simulink model "BLDC_speed_control"  (Simulink 8.1)
settings: Solver=ode45  StartTime=0.0  StopTime=1  RelTol=1e-3
InitFcn:
  | clc;
StopFcn:
  | clc;
undefined symbols (not defined in the file): emfg, Ts
libraries: simulink x6, powerlib x6, powerlib_extras x1
Description:
  | This simulink model simulates the speed control of permanent magnet
  | brush less DC motor. Complete dynamic model of brush-less DC motor
  | was developed and simulated. Conventional PI controller was employed
  | for speed loop.
  | 
  | Syed Abdul Rahman Kashif
  | EED, UET, Lahore
settings Model: Creator=AbdulRahman  LastModifiedBy=Sony
settings DataIOCC: SignalLoggingSaveFormat=Dataset
settings DebuggingCC: FcnCallInpInsideContextMsg=EnableAllAsError
settings GRTTargetCC: CombineOutputUpdateFcns=on  GRTInterface=off

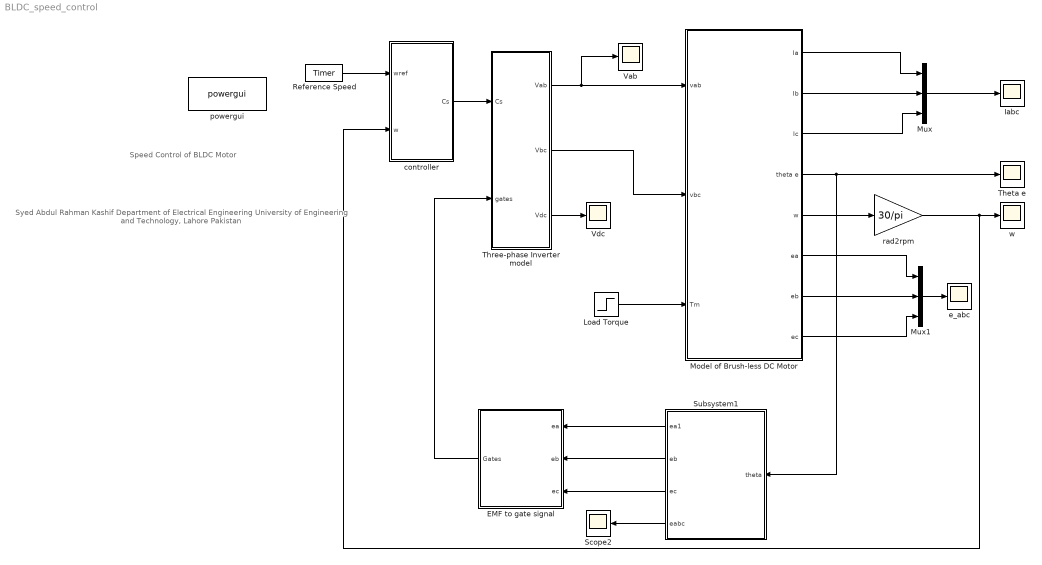
== system BLDC_speed_control ==
  note: Syed Abdul Rahman Kashif
      | Department of Electrical Engineering
      | University of Engineering and Technology, Lahore
      | Pakistan
  note: Speed Control of BLDC Motor
  EMF to gate signal : Subsystem
  Iabc : Scope
      settings: YMin=-0.3  YMax=0.3  SaveName=ScopeData4
  Load Torque : Step  Time=0.2  After=2  SampleTime=0
  Model of Brush-less DC Motor : Subsystem
  Mux : Mux  Inputs=3
  Mux1 : Mux  Inputs=3
  Reference Speed : powerlib_extras/Control  Blocks/Timer  t=[0 0.5]  e=[2000 1000]
  Scope2 : Scope
      settings: TimeRange=0.2  YMin=-2  YMax=2  SaveName=ScopeData2
  Subsystem1 : Subsystem
  Theta e : Scope
      settings: YMin=1.00059  YMax=1.00067
  Three-phase Inverter model : Subsystem
  Vab : Scope
      settings: TimeRange=0.2  YMin=-10000  YMax=10000  SaveName=ScopeData3
  Vdc : Scope
      settings: SaveName=ScopeData5
  controller : Subsystem
  e_abc : Scope
      settings: TimeRange=0.0001172995862488424  YMin=-150  YMax=150  SaveName=ScopeData6
  powergui : powerlib/powergui  Priority=2  SimulationMode=Continuous  SolverType=Tustin  SampleTime=Ts  frequency=60  SPID=off  DisableSnubberDevices=off  DisableRonSwitches=off  DisableVfSwitches=off  SwTol=0  Interpol=off  DisplayEquations=off  frequencyindice=0  Pbase=100e6  ErrMax=1e-4  Iterations=50  UnitsV=kV  UnitsW=MW  FunctionMessages=off  echomessages=off  HookPort=off  EnableUseOfTLC=off  x0status=blocks  RestoreLinks=warning  ResistiveCurrentMeasurement=off  Frange=[0:2:500]  Ylog=off  Xlog=on  ShowGrid=off  save=off  variable=ZData  ZoomFFT=on  StartTime=0.0  cycles=1  DisplayStyle=1  fundamental=60  FreqAxis=off  MaxFrequency=1000  frequencyindicesteady=1  RmsSteady=1  display=off  Ts=0  methode=off
  rad2rpm : Gain  Gain=30/pi
  w : Scope
      settings: TimeRange=0.4  YMin=0  YMax=2500
  wires:
  controller/1(Cs) -> Three-phase Inverter model/1(Cs)
  Three-phase Inverter model/2(Vbc) -> Model of Brush-less DC Motor/2(vbc)
  Three-phase Inverter model/3(Vdc) -> Vdc/1
  EMF to gate signal/1(Gates) -> Three-phase Inverter model/2(gates)
  Subsystem1/1(ea1) -> EMF to gate signal/1(ea)
  Subsystem1/2(eb) -> EMF to gate signal/2(eb)
  Subsystem1/3(ec) -> EMF to gate signal/3(ec)
  Model of Brush-less DC Motor/4(theta e) -> Theta e/1, Subsystem1/1(theta)
  Load Torque/1 -> Model of Brush-less DC Motor/3(Tm)
  Model of Brush-less DC Motor/2(Ib) -> Mux/2
  Model of Brush-less DC Motor/3(Ic) -> Mux/3
  Model of Brush-less DC Motor/6(ea) -> Mux1/1
  Model of Brush-less DC Motor/7(eb) -> Mux1/2
  Model of Brush-less DC Motor/8(ec) -> Mux1/3
  Mux1/1 -> e_abc/1
  Subsystem1/4(eabc) -> Scope2/1
  Model of Brush-less DC Motor/5(w) -> rad2rpm/1
  rad2rpm/1 -> controller/2(w), w/1
  Model of Brush-less DC Motor/1(Ia) -> Mux/1
  Mux/1 -> Iabc/1
  Reference Speed/1 -> controller/1(wref)
  Three-phase Inverter model/1(Vab) -> Model of Brush-less DC Motor/1(vab), Vab/1

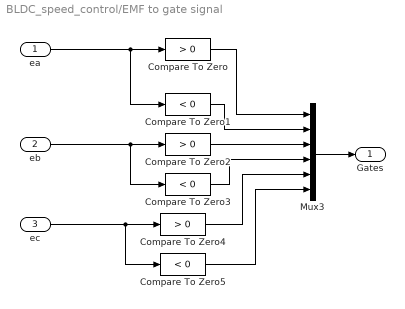
== system BLDC_speed_control/EMF to gate signal ==
  ea : Inport
  eb : Inport  Port=2
  ec : Inport  Port=3
  Compare To Zero : simulink/Logic and Bit Operations/Compare To Zero  relop=>  OutDataTypeStr=boolean  ZeroCross=off
  Compare To Zero1 : simulink/Logic and Bit Operations/Compare To Zero  relop=<  OutDataTypeStr=boolean  ZeroCross=off
  Compare To Zero2 : simulink/Logic and Bit Operations/Compare To Zero  relop=>  OutDataTypeStr=boolean  ZeroCross=off
  Compare To Zero3 : simulink/Logic and Bit Operations/Compare To Zero  relop=<  OutDataTypeStr=boolean  ZeroCross=off
  Compare To Zero4 : simulink/Logic and Bit Operations/Compare To Zero  relop=>  OutDataTypeStr=boolean  ZeroCross=off
  Compare To Zero5 : simulink/Logic and Bit Operations/Compare To Zero  relop=<  OutDataTypeStr=boolean  ZeroCross=off
  Mux3 : Mux  Inputs=6
  Gates : Outport
  wires:
  Mux3/1 -> Gates/1
  ea/1 -> Compare To Zero/1, Compare To Zero1/1
  eb/1 -> Compare To Zero2/1, Compare To Zero3/1
  ec/1 -> Compare To Zero4/1, Compare To Zero5/1
  Compare To Zero/1 -> Mux3/1
  Compare To Zero1/1 -> Mux3/2
  Compare To Zero2/1 -> Mux3/3
  Compare To Zero3/1 -> Mux3/4
  Compare To Zero4/1 -> Mux3/5
  Compare To Zero5/1 -> Mux3/6

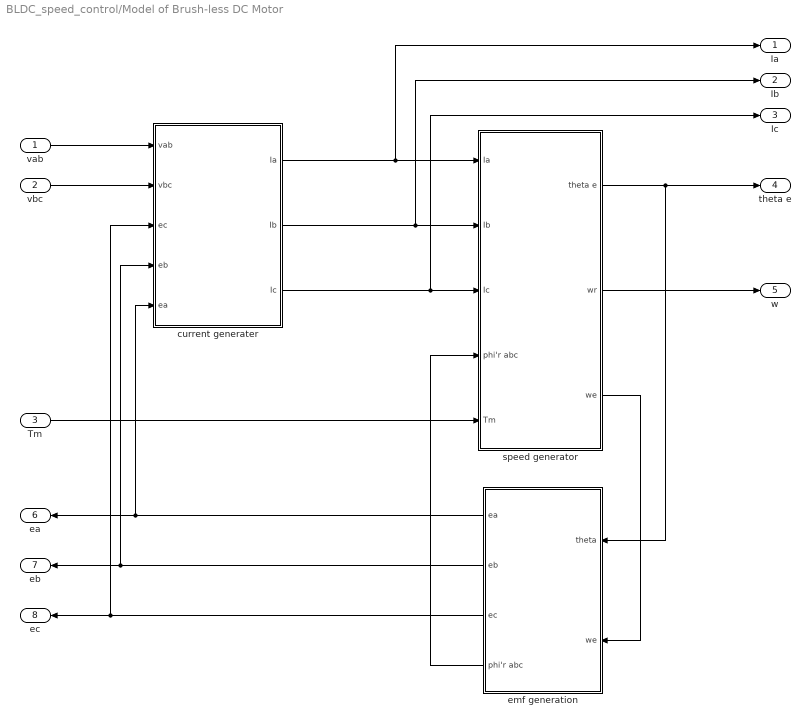
== system BLDC_speed_control/Model of Brush-less DC Motor ==
  vab : Inport
  vbc : Inport  Port=2
  Tm : Inport  Port=3
  current generater : Subsystem
  emf generation : Subsystem
  speed generator : Subsystem
  Ia : Outport
  Ib : Outport  Port=2
  Ic : Outport  Port=3
  theta e : Outport  Port=4
  w : Outport  Port=5
  ea : Outport  Port=6
  eb : Outport  Port=7
  ec : Outport  Port=8
  wires:
  vab/1 -> current generater/1(vab)
  vbc/1 -> current generater/2(vbc)
  current generater/1(Ia) -> Ia/1, speed generator/1(Ia)
  current generater/2(Ib) -> Ib/1, speed generator/2(Ib)
  current generater/3(Ic) -> speed generator/3(Ic), Ic/1
  speed generator/1(theta e) -> emf generation/1(theta), theta e/1
  Tm/1 -> speed generator/5(Tm)
  speed generator/2(wr) -> w/1
  emf generation/1(ea) -> ea/1, current generater/5(ea)
  emf generation/2(eb) -> eb/1, current generater/4(eb)
  emf generation/3(ec) -> ec/1, current generater/3(ec)
  emf generation/4(phi'r abc) -> speed generator/4(phi'r abc)
  speed generator/3(we) -> emf generation/2(we)

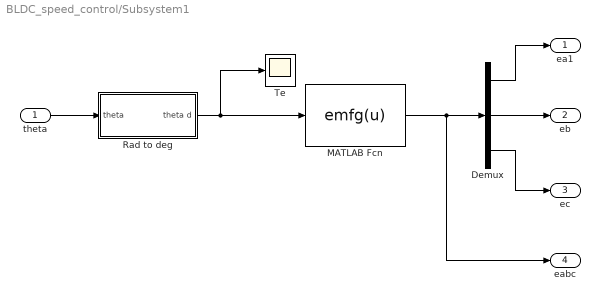
== system BLDC_speed_control/Subsystem1 ==
  theta : Inport
  Demux : Demux  Outputs=3
  MATLAB Fcn : MATLABFcn  MATLABFcn=emfg(u)  OutputDimensions=3
  Rad to deg : Subsystem
  Te : Scope
      settings: TimeRange=0.0001172995862488424  YMin=-200  YMax=200  SaveName=ScopeData12
  ea1 : Outport
  eb : Outport  Port=2
  ec : Outport  Port=3
  eabc : Outport  Port=4
  wires:
  Demux/1 -> ea1/1
  Demux/2 -> eb/1
  Demux/3 -> ec/1
  theta/1 -> Rad to deg/1(theta)
  Rad to deg/1(theta d) -> MATLAB Fcn/1, Te/1
  MATLAB Fcn/1 -> eabc/1, Demux/1

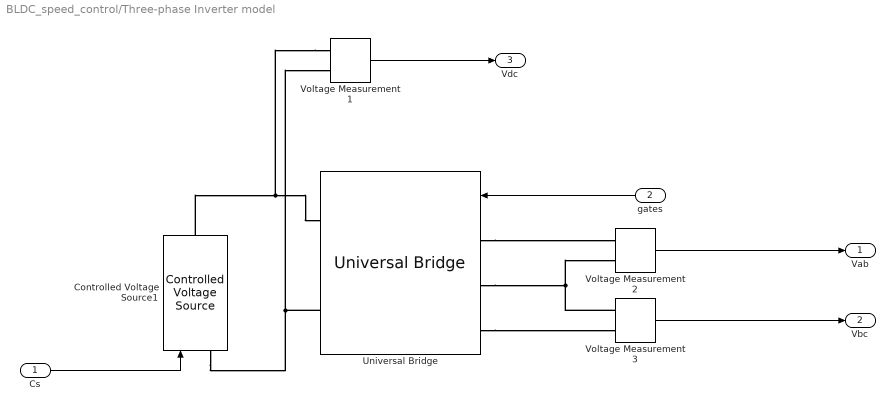
== system BLDC_speed_control/Three-phase Inverter model ==
  Cs : Inport
  gates : Inport  Port=2
  Controlled Voltage Source1 : powerlib/Electrical Sources/Controlled Voltage Source  Initialize=on  Source_Type=AC  Amplitude=500  Phase=0  Frequency=0  Measurements=None
  Universal Bridge : powerlib/Power Electronics/Universal Bridge  Arms=3  SnubberResistance=5000  SnubberCapacitance=1e-6  Device=MOSFET / Diodes  Ron=1e-3  Lon=0  ForwardVoltages="[  0  0  ]"  ForwardVoltage=0  GTOparameters=[ 10e-6 , 20e-6 ]  IGBTparameters=[ 1e-6 , 2e-6 ]  Measurements=None  Measurements_2=None  converterType=Rectifier
  Voltage Measurement1 : powerlib/Measurements/Voltage Measurement  PhasorSimulation=off  OutputType=Complex  PSBequivalent=0
  Voltage Measurement2 : powerlib/Measurements/Voltage Measurement  PhasorSimulation=off  OutputType=Complex  PSBequivalent=0
      link override source: GotoTag=tp96803dc0_013b_4907_89cd_69d70f818148
  Voltage Measurement3 : powerlib/Measurements/Voltage Measurement  PhasorSimulation=off  OutputType=Complex  PSBequivalent=0
  Vab : Outport
  Vbc : Outport  Port=2
  Vdc : Outport  Port=3
  wires:
  Cs/1 -> Controlled Voltage Source1/1
  gates/1 -> Universal Bridge/1
  Voltage Measurement1/1 -> Vdc/1
  Voltage Measurement2/1 -> Vab/1
  Voltage Measurement3/1 -> Vbc/1
  connections:
  Voltage Measurement1/LConn1 -- Controlled Voltage Source1/RConn1 -- Universal Bridge/RConn1
  Controlled Voltage Source1/LConn1 -- Voltage Measurement1/LConn2 -- Universal Bridge/RConn2
  Universal Bridge/LConn1 -- Voltage Measurement2/LConn1
  Voltage Measurement3/LConn1 -- Voltage Measurement2/LConn2 -- Universal Bridge/LConn2
  Universal Bridge/LConn3 -- Voltage Measurement3/LConn2

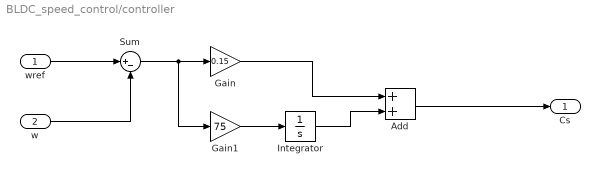
== system BLDC_speed_control/controller ==
  wref : Inport
  w : Inport  Port=2
  Add : Sum
  Gain : Gain  Gain=0.15
  Gain1 : Gain  Gain=75
  Integrator : Integrator
  Sum : Sum  Inputs=|+-
  Cs : Outport
  wires:
  wref/1 -> Sum/1
  w/1 -> Sum/2
  Sum/1 -> Gain1/1, Gain/1
  Add/1 -> Cs/1
  Gain1/1 -> Integrator/1
  Gain/1 -> Add/1
  Integrator/1 -> Add/2

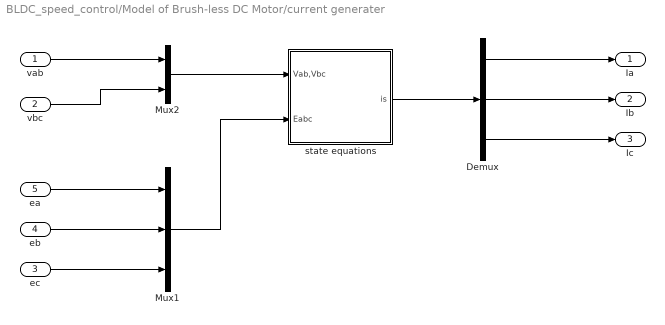
== system BLDC_speed_control/Model of Brush-less DC Motor/current generater ==
  vab : Inport
  vbc : Inport  Port=2
  ec : Inport  Port=3
  eb : Inport  Port=4
  ea : Inport  Port=5
  Demux : Demux  Outputs=3
  Mux1 : Mux  Inputs=3
  Mux2 : Mux  Inputs=2
  state equations : Subsystem
  Ia : Outport
  Ib : Outport  Port=2
  Ic : Outport  Port=3
  wires:
  state equations/1(is) -> Demux/1
  ea/1 -> Mux1/1
  eb/1 -> Mux1/2
  ec/1 -> Mux1/3
  Mux1/1 -> state equations/2(Eabc)
  Demux/1 -> Ia/1
  Demux/2 -> Ib/1
  Demux/3 -> Ic/1
  vab/1 -> Mux2/1
  vbc/1 -> Mux2/2
  Mux2/1 -> state equations/1(Vab,Vbc)

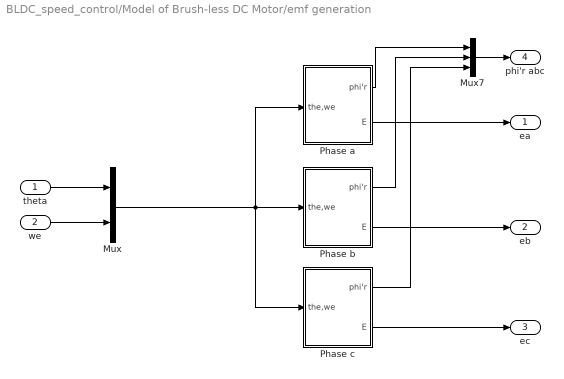
== system BLDC_speed_control/Model of Brush-less DC Motor/emf generation ==
  theta : Inport
  we : Inport  Port=2
  Mux : Mux  Inputs=2
  Mux7 : Mux  Inputs=3
  Phase a : Subsystem
  Phase b : Subsystem
  Phase c : Subsystem
  ea : Outport
  eb : Outport  Port=2
  ec : Outport  Port=3
  phi'r abc : Outport  Port=4
  wires:
  Mux7/1 -> phi'r abc/1
  Phase c/1(phi'r) -> Mux7/3
  Phase b/1(phi'r) -> Mux7/2
  Phase a/1(phi'r) -> Mux7/1
  Mux/1 -> Phase a/1(the,we), Phase b/1(the,we), Phase c/1(the,we)
  Phase a/2(E) -> ea/1
  Phase b/2(E) -> eb/1
  Phase c/2(E) -> ec/1
  theta/1 -> Mux/1
  we/1 -> Mux/2

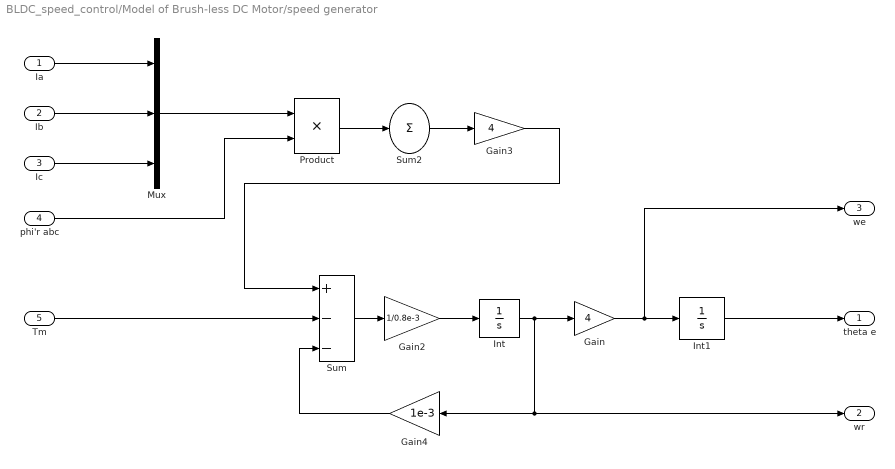
== system BLDC_speed_control/Model of Brush-less DC Motor/speed generator ==
  Ia : Inport
  Ib : Inport  Port=2
  Ic : Inport  Port=3
  phi'r abc : Inport  Port=4
  Tm : Inport  Port=5
  Gain : Gain  Gain=4  SaturateOnIntegerOverflow=on  OutDataTypeStr=Inherit: Same as input  ParamDataTypeStr=Inherit: Same as input
  Gain2 : Gain  Gain=1/0.8e-3  SaturateOnIntegerOverflow=on  OutDataTypeStr=Inherit: Same as input  ParamDataTypeStr=Inherit: Same as input
  Gain3 : Gain  Gain=4  SaturateOnIntegerOverflow=on  OutDataTypeStr=Inherit: Same as input  ParamDataTypeStr=Inherit: Same as input
  Gain4 : Gain  Gain=1e-3  SaturateOnIntegerOverflow=on  OutDataTypeStr=Inherit: Same as input  ParamDataTypeStr=Inherit: Same as input
  Int : Integrator
  Int1 : Integrator
  Mux : Mux  Inputs=3
  Product : Product  SaturateOnIntegerOverflow=on  OutDataTypeStr=Inherit: Same as first input
  Sum : Sum  Inputs=+--  SaturateOnIntegerOverflow=on  InputSameDT=on  OutDataTypeStr=Inherit: Same as first input
  Sum2 : Sum  Inputs=+  SaturateOnIntegerOverflow=on
  theta e : Outport
  wr : Outport  Port=2
  we : Outport  Port=3
  wires:
  Ia/1 -> Mux/1
  Ib/1 -> Mux/2
  Ic/1 -> Mux/3
  Gain3/1 -> Sum/1
  Sum2/1 -> Gain3/1
  Product/1 -> Sum2/1
  Mux/1 -> Product/1
  phi'r abc/1 -> Product/2
  Int1/1 -> theta e/1
  Gain/1 -> Int1/1, we/1
  Int/1 -> Gain/1, Gain4/1, wr/1
  Gain2/1 -> Int/1
  Sum/1 -> Gain2/1
  Gain4/1 -> Sum/3
  Tm/1 -> Sum/2

== system BLDC_speed_control/Subsystem1/Rad to deg ==
  theta : Inport
  Trigonometric Function : Trigonometry
  Trigonometric Function1 : Trigonometry  Operator=cos
  Trigonometric Function2 : Trigonometry  Operator=atan2
  rad2deg : Gain  Gain=180/pi  SaturateOnIntegerOverflow=on  OutDataTypeStr=Inherit: Same as input  ParamDataTypeStr=Inherit: Same as input
  theta d : Outport
  wires:
  theta/1 -> Trigonometric Function/1, Trigonometric Function1/1
  Trigonometric Function/1 -> Trigonometric Function2/1
  Trigonometric Function1/1 -> Trigonometric Function2/2
  Trigonometric Function2/1 -> rad2deg/1
  rad2deg/1 -> theta d/1

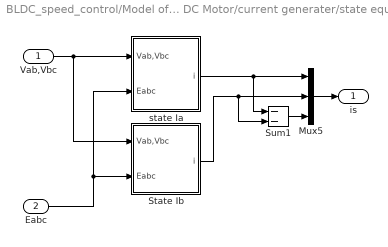
== system BLDC_speed_control/Model of Brush-less DC Motor/current generater/state equations ==
  Vab,Vbc : Inport
  Eabc : Inport  Port=2
  Mux5 : Mux  Inputs=3
  State Ib : Subsystem
  Sum1 : Sum  Inputs=--  SaturateOnIntegerOverflow=on
  state Ia : Subsystem
  is : Outport
  wires:
  Mux5/1 -> is/1
  Eabc/1 -> state Ia/2(Eabc), State Ib/2(Eabc)
  Sum1/1 -> Mux5/3
  State Ib/1(i) -> Sum1/2, Mux5/2
  state Ia/1(i) -> Sum1/1, Mux5/1
  Vab,Vbc/1 -> state Ia/1(Vab,Vbc), State Ib/1(Vab,Vbc)

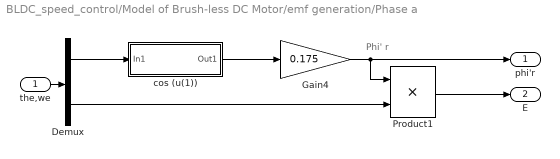
== system BLDC_speed_control/Model of Brush-less DC Motor/emf generation/Phase a ==
  note: Phi' r
  the,we : Inport
  Demux : Demux  Outputs=2
  Gain4 : Gain  Gain=0.175  SaturateOnIntegerOverflow=on  OutDataTypeStr=Inherit: Same as input  ParamDataTypeStr=Inherit: Same as input
  Product1 : Product  SaturateOnIntegerOverflow=on  OutDataTypeStr=Inherit: Same as first input
  cos (u(1)) : Subsystem
  phi'r : Outport
  E : Outport  Port=2
  wires:
  Gain4/1 -> Product1/1, phi'r/1
  Product1/1 -> E/1
  the,we/1 -> Demux/1
  Demux/2 -> Product1/2
  Demux/1 -> cos (u(1))/1(In1)
  cos (u(1))/1(Out1) -> Gain4/1

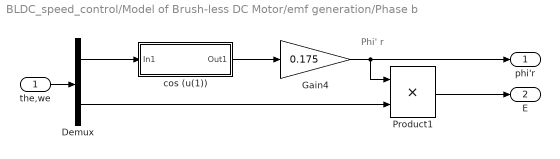
== system BLDC_speed_control/Model of Brush-less DC Motor/emf generation/Phase b ==
  note: Phi' r
  the,we : Inport
  Demux : Demux  Outputs=2
  Gain4 : Gain  Gain=0.175  SaturateOnIntegerOverflow=on  OutDataTypeStr=Inherit: Same as input  ParamDataTypeStr=Inherit: Same as input
  Product1 : Product  SaturateOnIntegerOverflow=on  OutDataTypeStr=Inherit: Same as first input
  cos (u(1)) : Subsystem
  phi'r : Outport
  E : Outport  Port=2
  wires:
  cos (u(1))/1(Out1) -> Gain4/1
  Demux/1 -> cos (u(1))/1(In1)
  Demux/2 -> Product1/2
  the,we/1 -> Demux/1
  Product1/1 -> E/1
  Gain4/1 -> phi'r/1, Product1/1

== system BLDC_speed_control/Model of Brush-less DC Motor/emf generation/Phase c ==
  note: Phi' r
  the,we : Inport
  Demux : Demux  Outputs=2
  Gain4 : Gain  Gain=0.175  SaturateOnIntegerOverflow=on  OutDataTypeStr=Inherit: Same as input  ParamDataTypeStr=Inherit: Same as input
  Product1 : Product  SaturateOnIntegerOverflow=on  OutDataTypeStr=Inherit: Same as first input
  cos (u(1)) : Subsystem
  phi'r : Outport
  E : Outport  Port=2
  wires:
  Gain4/1 -> Product1/1, phi'r/1
  Product1/1 -> E/1
  the,we/1 -> Demux/1
  Demux/2 -> Product1/2
  Demux/1 -> cos (u(1))/1(In1)
  cos (u(1))/1(Out1) -> Gain4/1

== system BLDC_speed_control/Model of Brush-less DC Motor/current generater/state equations/State Ib ==
  Vab,Vbc : Inport
  Eabc : Inport  Port=2
  Fcn : Fcn  Expr=-u(1)+u(2)+u(3)-2*u(4)+u(5)-3*2.8750*u(6)
  Gain2 : Gain  Gain=1/(3*.0085)  SaturateOnIntegerOverflow=on  OutDataTypeStr=Inherit: Same as input  ParamDataTypeStr=Inherit: Same as input
  Mux : Mux  Inputs=3
  "s " : Integrator
  i : Outport
  wires:
  Gain2/1 -> "s "/1
  Vab,Vbc/1 -> Mux/1
  Eabc/1 -> Mux/2
  Mux/1 -> Fcn/1
  Fcn/1 -> Gain2/1
  "s "/1 -> Mux/3, i/1

== system BLDC_speed_control/Model of Brush-less DC Motor/current generater/state equations/state Ia ==
  Vab,Vbc : Inport
  Eabc : Inport  Port=2
  Fcn : Fcn  Expr=2*u(1)+u(2)-2*u(3)+u(4)+u(5)-3*2.8750*u(6)
  Gain2 : Gain  Gain=1/(3*.0085)  SaturateOnIntegerOverflow=on  OutDataTypeStr=Inherit: Same as input  ParamDataTypeStr=Inherit: Same as input
  Mux : Mux  Inputs=3
  "s " : Integrator
  i : Outport
  wires:
  "s "/1 -> Mux/3, i/1
  Fcn/1 -> Gain2/1
  Mux/1 -> Fcn/1
  Eabc/1 -> Mux/2
  Vab,Vbc/1 -> Mux/1
  Gain2/1 -> "s "/1

== system BLDC_speed_control/Model of Brush-less DC Motor/emf generation/Phase a/cos (u(1)) ==
  In1 : Inport
  Fcn : Fcn  Expr=cos(u(1))
  Saturation : Saturate  UpperLimit=0.8  LowerLimit=-0.8
  Out1 : Outport
  wires:
  In1/1 -> Fcn/1
  Fcn/1 -> Saturation/1
  Saturation/1 -> Out1/1

== system BLDC_speed_control/Model of Brush-less DC Motor/emf generation/Phase b/cos (u(1)) ==
  In1 : Inport
  Fcn : Fcn  Expr=cos(u(1)-2*pi/3)
  Saturation : Saturate  UpperLimit=0.8  LowerLimit=-0.8
  Out1 : Outport
  wires:
  In1/1 -> Fcn/1
  Fcn/1 -> Saturation/1
  Saturation/1 -> Out1/1

== system BLDC_speed_control/Model of Brush-less DC Motor/emf generation/Phase c/cos (u(1)) ==
  In1 : Inport
  Fcn1 : Fcn  Expr=cos(u(1)+2*pi/3)
  Saturation : Saturate  UpperLimit=0.8  LowerLimit=-0.8
  Out1 : Outport
  wires:
  In1/1 -> Fcn1/1
  Fcn1/1 -> Saturation/1
  Saturation/1 -> Out1/1
